simulink model "IDTmodel"  (R2021a)
settings: Solver=ode23tb  StartTime=0.0  StopTime=0.75  FixedStep=4e-4  RelTol=1e-3  EnableMultiTasking=on
PreLoadFcn:
  | % -- Recommended Settings --
  | %
  | %  Simulink:
  | %      Solver: Ode23tb
  | %      Relative tolerance = 1e-4
  | %      Max step size = 0.2
  | %
  | %  Powergui:
  |          Ts = 1e-06; % (discrete electrical model)
  | %
  | %  Control systems:
  |          Ts_control = 10*Ts; % (discrete control system)
  | %
  | % ----------------------------------
InitFcn:
  | Ts=1e-5;
  | Ts_control=1e-5;
undefined symbols (not defined in the file or in its folder): D1, Delta
libraries: spsThreePhaseVIMeasurementLib x26, spsThreePhaseSeriesRLCLoadLib x8, spsabctoAlphaBetaZeroLib x6, spsThreePhaseSeriesRLCBranchLib x6, spsThreePhaseTransformerTwoWindingsLib x5, spsDistributedParametersLineLib x5, spsPowerPositiveSequenceLib x4, spsThreePhaseBreakerLib x4, spsDCVoltageSourceLib x2, spsSVPWMGenerator2LevelLib x2, spsGroundLib x2, spsUniversalBridgeLib x2
(part 1 of 2)
settings Model: Creator=Basit Bukhari  LastModifiedBy=Dell
settings DataIOCC: InitialState=x0  LimitDataPoints=on  ReturnWorkspaceOutputs=off  Refine=10
settings OptimizationCC: EfficientMapNaN2IntZero=off  LifeSpan=inf
settings DebuggingCC: UnconnectedInputMsg=none  UnconnectedOutputMsg=none  UnconnectedLineMsg=none  AllowSymbolicDim=off  SFUnexpectedBacktrackingDiag=warning  SFNoUnconditionalDefaultTransitionDiag=warning  SFExecutionAtInitializationDiag=none  SFMachineParentedDataDiag=warning  ArithmeticOperatorsInVariantConditions=warning
settings HardwareCC: TargetBitPerPointer=64  TargetBitPerSizeT=64  TargetBitPerPtrDiffT=64  TargetLongLongMode=on  TargetIntDivRoundTo=Zero  TargetEndianess=LittleEndian  TargetWordSize=64  TargetHWDeviceType=MATLAB Host  ProdEqTarget=off
settings SFSimCC: SimUseLocalCustomCode=off  CustomCodeUndefinedFunction=UseInterfaceOnly
settings RTWCC: RTWUseLocalCustomCode=off
settings CodeAppCC: MaxIdLength=128
settings GRTTargetCC: TargetLangStandard=C89/C90 (ANSI)  CombineOutputUpdateFcns=off  GRTInterface=on
settings ConfigComp: CovMetricSettings=dw  CovSaveCumulativeToWorkspaceVar=on  CovSaveSingleToWorkspaceVar=on  CovExternalEMLEnable=off  CovSFcnEnable=off
settings SimscapeCC: SimscapeNormalizeSystem=off

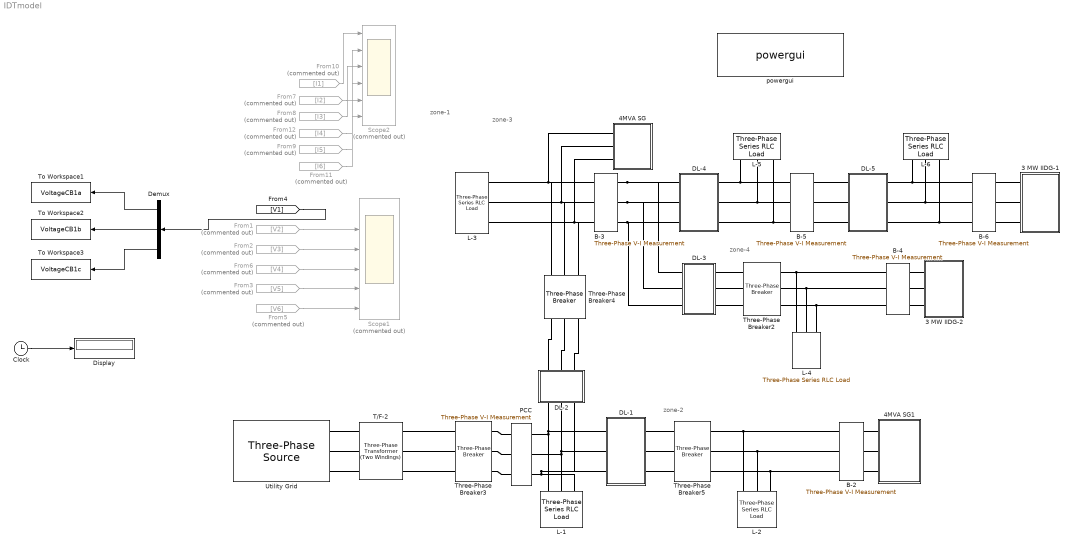
== system IDTmodel ==
  note: zone-2
  note: zone-3
  note: zone-1
  note: zone-4
  " B-2" : spsThreePhaseVIMeasurementLib/Three-Phase V-I Measurement  VoltageMeasurement=phase-to-ground  SetLabelV=on  LabelV=V2  Vpu=on  VpuLL=off  CurrentMeasurement=yes  SetLabelI=on  LabelI=I2  Ipu=on  Pbase=10e6  Vbase=25e3  OutputType=Magnitude  PhasorSimulation=off  PSBequivalent=0
  " B-3" : spsThreePhaseVIMeasurementLib/Three-Phase V-I Measurement  VoltageMeasurement=phase-to-ground  SetLabelV=on  LabelV=V3  Vpu=on  VpuLL=off  CurrentMeasurement=yes  SetLabelI=on  LabelI=I3  Ipu=on  Pbase=10e6  Vbase=25e3  OutputType=Magnitude  PhasorSimulation=off  PSBequivalent=0
  " B-4" : spsThreePhaseVIMeasurementLib/Three-Phase V-I Measurement  VoltageMeasurement=phase-to-ground  SetLabelV=on  LabelV=V4  Vpu=on  VpuLL=off  CurrentMeasurement=yes  SetLabelI=on  LabelI=I4  Ipu=on  Pbase=10e6  Vbase=25e3  OutputType=Magnitude  PhasorSimulation=off  PSBequivalent=0
  " B-5" : spsThreePhaseVIMeasurementLib/Three-Phase V-I Measurement  VoltageMeasurement=phase-to-ground  SetLabelV=on  LabelV=V5  Vpu=on  VpuLL=off  CurrentMeasurement=yes  SetLabelI=on  LabelI=I5  Ipu=on  Pbase=10e6  Vbase=25e3  OutputType=Magnitude  PhasorSimulation=off  PSBequivalent=0
  " B-6" : spsThreePhaseVIMeasurementLib/Three-Phase V-I Measurement  VoltageMeasurement=phase-to-ground  SetLabelV=on  LabelV=V6  Vpu=on  VpuLL=off  CurrentMeasurement=yes  SetLabelI=on  LabelI=I6  Ipu=on  Pbase=10e6  Vbase=25e3  OutputType=Magnitude  PhasorSimulation=off  PSBequivalent=0
  " PCC" : spsThreePhaseVIMeasurementLib/Three-Phase V-I Measurement  VoltageMeasurement=phase-to-ground  SetLabelV=on  LabelV=V1  Vpu=on  VpuLL=off  CurrentMeasurement=yes  SetLabelI=on  LabelI=I1  Ipu=on  Pbase=10e6  Vbase=25e3  OutputType=Magnitude  PhasorSimulation=off  PSBequivalent=0
  3 MW IIDG-1 : Subsystem
  3 MW IIDG-2 : Subsystem
  4MVA SG : Subsystem
  4MVA SG1 : Subsystem
  Clock : Clock
  DL-1 : Subsystem
  DL-2 : Subsystem
  DL-3 : Subsystem
  DL-4 : Subsystem
  DL-5 : Subsystem
  Demux : Demux  Outputs=3
  Display : Display
  From1 : From  Commented=on  GotoTag=V2  TagVisibility=global
  From10 : From  Commented=on  GotoTag=I1  TagVisibility=global
  From11 : From  Commented=on  GotoTag=I6  TagVisibility=global
  From12 : From  Commented=on  GotoTag=I4  TagVisibility=global
  From2 : From  Commented=on  GotoTag=V3  TagVisibility=global
  From3 : From  Commented=on  GotoTag=V5  TagVisibility=global
  From5 : From  Commented=on  GotoTag=V6  TagVisibility=global
  From6 : From  Commented=on  GotoTag=V4  TagVisibility=global
  From7 : From  Commented=on  GotoTag=I2  TagVisibility=global
  From8 : From  Commented=on  GotoTag=I3  TagVisibility=global
  From9 : From  Commented=on  GotoTag=I5  TagVisibility=global
  L-1 : spsThreePhaseSeriesRLCLoadLib/Three-Phase Series RLC Load  LConnTagsString=A|B|C  Configuration=Y (grounded)  NominalVoltage=25e3  Vabc=[7.2 7.2 7.2]*1e3  Vabcp=[1e3 1e3 1e3]  NominalFrequency=50  UnbalancedPower=off  ActivePower=1.5e6  InductivePower=0.6e6  CapacitivePower=0  Pabc=[250 300 350]*1e3  QLabc=[136 170 220]*1e3  QCabc=[0 0 0]  Pabcp=[10e3 9e3 11e3]  QLabcp=[100 90 110]  QCabcp=[100 90 110]  Measurements=None  LoadType=constant PQ
  L-2 : spsThreePhaseSeriesRLCLoadLib/Three-Phase Series RLC Load  LConnTagsString=A|B|C  Configuration=Y (grounded)  NominalVoltage=25e3  Vabc=[7.2 7.2 7.2]*1e3  Vabcp=[1e3 1e3 1e3]  NominalFrequency=50  UnbalancedPower=off  ActivePower=1.5e6  InductivePower=0.3e6  CapacitivePower=0  Pabc=[250 300 350]*1e3  QLabc=[136 170 220]*1e3  QCabc=[0 0 0]  Pabcp=[10e3 9e3 11e3]  QLabcp=[100 90 110]  QCabcp=[100 90 110]  Measurements=None  LoadType=constant PQ
  L-3 : spsThreePhaseSeriesRLCLoadLib/Three-Phase Series RLC Load  LConnTagsString=A|B|C  Configuration=Y (grounded)  NominalVoltage=25e3  Vabc=[7.2 7.2 7.2]*1e3  Vabcp=[1e3 1e3 1e3]  NominalFrequency=50  UnbalancedPower=off  ActivePower=1e6  InductivePower=0.2e6  CapacitivePower=0  Pabc=[250 300 350]*1e3  QLabc=[136 170 220]*1e3  QCabc=[0 0 0]  Pabcp=[10e3 9e3 11e3]  QLabcp=[100 90 110]  QCabcp=[100 90 110]  Measurements=None  LoadType=constant Z
  L-4 : spsThreePhaseSeriesRLCLoadLib/Three-Phase Series RLC Load  LConnTagsString=A|B|C  Configuration=Y (grounded)  NominalVoltage=25e3  Vabc=[7.2 7.2 7.2]*1e3  Vabcp=[1e3 1e3 1e3]  NominalFrequency=50  UnbalancedPower=off  ActivePower=1.5e6  InductivePower=0.6e6  CapacitivePower=0  Pabc=[250 300 350]*1e3  QLabc=[136 170 220]*1e3  QCabc=[0 0 0]  Pabcp=[10e3 9e3 11e3]  QLabcp=[100 90 110]  QCabcp=[100 90 110]  Measurements=None  LoadType=constant Z
  L-5 : spsThreePhaseSeriesRLCLoadLib/Three-Phase Series RLC Load  LConnTagsString=A|B|C  Configuration=Y (grounded)  NominalVoltage=25e3  Vabc=[7.2 7.2 7.2]*1e3  Vabcp=[1e3 1e3 1e3]  NominalFrequency=50  UnbalancedPower=off  ActivePower=0.5e6  InductivePower=0.1e6  CapacitivePower=0  Pabc=[250 300 350]*1e3  QLabc=[136 170 220]*1e3  QCabc=[0 0 0]  Pabcp=[10e3 9e3 11e3]  QLabcp=[100 90 110]  QCabcp=[100 90 110]  Measurements=None  LoadType=constant Z
  L-6 : spsThreePhaseSeriesRLCLoadLib/Three-Phase Series RLC Load  LConnTagsString=A|B|C  Configuration=Y (grounded)  NominalVoltage=25e3  Vabc=[7.2 7.2 7.2]*1e3  Vabcp=[1e3 1e3 1e3]  NominalFrequency=50  UnbalancedPower=off  ActivePower=1e6  InductivePower=0.3e6  CapacitivePower=0  Pabc=[250 300 350]*1e3  QLabc=[136 170 220]*1e3  QCabc=[0 0 0]  Pabcp=[10e3 9e3 11e3]  QLabcp=[100 90 110]  QCabcp=[100 90 110]  Measurements=None  LoadType=constant Z
  Scope1 : Scope  Commented=on  NumInputPorts=6
  Scope2 : Scope  Commented=on  NumInputPorts=6
  T/F-2 : spsThreePhaseTransformerTwoWindingsLib/Three-Phase Transformer (Two Windings)  Winding1Connection=Delta (D1)  Winding2Connection=Yg  CoreType=Three single-phase transformers  SetSaturation=off  Hysteresis=off  DataFile='hysteresis'  SetInitialFlux=off  Measurements=None  UNITS=pu  NominalPower=[20e6 , 50 ]  Winding1=[120e3 , 0.00375 , 0.1]  Winding2=[25e3 , 0.00375 , 0.1]  Rm=500  Lm=500  L0=0.5  Saturation=[ 0,0 ; 0.0024,1.2 ; 1.0,1.52 ]  InitialFluxes=[ 0.8 , -0.8 , 0.7 ]  BreakLoop=off  DiscreteSolver=Trapezoidal iterative  DataType=off  TransfoNumber=1
  Three-Phase Breaker{2..5} (4 alike) : spsThreePhaseBreakerLib/Three-Phase Breaker  InitialState=closed  SwitchA=on  SwitchB=on  SwitchC=on  SwitchTimes=[5]  External=off  BreakerResistance=0.01  SnubberResistance=1e6  SnubberCapacitance=inf  Measurements=None
  To Workspace1 : ToWorkspace  VariableName=VoltageCB1a  SaveFormat=Timeseries  SampleTime=1/3840
  To Workspace2 : ToWorkspace  VariableName=VoltageCB1b  SaveFormat=Timeseries  SampleTime=1/3840
  To Workspace3 : ToWorkspace  VariableName=VoltageCB1c  SaveFormat=Timeseries  SampleTime=1/3840
  "Utility Grid  " : spsThreePhaseSourceLib/Three-Phase Source  InternalConnection=Yg  VoltagePhases=off  Voltage=120e3  PhaseAngle=0  Voltage_phases=[25e3 25e3 25e3]/sqrt(3)  PhaseAngles_phases=[0 -120 +120]  Frequency=50  NonIdealSource=on  SpecifyImpedance=on  Resistance=0.8929  Inductance=16.58e-3  ShortCircuitLevel=500e6  BaseVoltage=120e3  XRratio=7  BusType=swing  Pref=10e6  Qref=5e6  Prefabc=[10e3, 10e3, 10e3]  Qrefabc=[0, 0, 0]  Qmin=-inf  Qmax=inf
  powergui : spspowerguiLib/powergui  Priority=1  SimulationMode=Discrete  SampleTime=10e-6  frequency=60  Iterations=50  frequencyindice=50  Pbase=100e6  ErrMax=1e-4  UnitsV=kV  UnitsW=MW  buscounter=0  FunctionMessages=off  echomessages=off  EnableUseOfTLC=off  CurrentSourceSwitches=off  DisableSnubberDevices=off  DisableRonSwitches=off  DisableVfSwitches=off  DisplayEquations=off  AutomaticDiscreteSolvers=off  SolverType=Tustin/Backward Euler (TBE)  Interpol=off  ExternalGateDelay=off  methode=off  Ts=100  x0status=steady  SPID=on  SwTol=0  HookPort=off  NonlinearTolerance=1e-4  nMaxIteration=100  ContinueOnMaxIteration=off  RestoreLinks=warning  ResistiveCurrentMeasurement=off  Frange=[0:2:500]  Ylog=off  Xlog=on  ShowGrid=off  save=off  variable=ZData  structure=0  ZoomFFT=off  StartTime=0.0  cycles=1  DisplayStyle=1  fundamental=60  FreqAxis=off  MaxFrequency=1000  frequencyindicesteady=1  RmsSteady=1  display=off
  wires:
  From9/1 -> Scope2/5
  From8/1 -> Scope2/3
  From7/1 -> Scope2/2
  From10/1 -> Scope2/1
  From12/1 -> Scope2/4
  From11/1 -> Scope2/6
  Demux/2 -> To Workspace2/1
  Demux/1 -> To Workspace1/1
  Demux/3 -> To Workspace3/1
  From3/1 -> Scope1/5
  From2/1 -> Scope1/3
  From6/1 -> Scope1/4
  [V1] -> Demux/1
  From5/1 -> Scope1/6
  From1/1 -> Scope1/2
  Clock/1 -> Display/1
  connections:
  T/F-2/LConn1 -- "Utility Grid  "/RConn1
  T/F-2/LConn2 -- "Utility Grid  "/RConn2
  T/F-2/LConn3 -- "Utility Grid  "/RConn3
  Three-Phase Breaker3/LConn1 -- T/F-2/RConn1
  Three-Phase Breaker3/LConn2 -- T/F-2/RConn2
  Three-Phase Breaker3/LConn3 -- T/F-2/RConn3
  " PCC"/LConn1 -- Three-Phase Breaker3/RConn1
  " PCC"/LConn2 -- Three-Phase Breaker3/RConn2
  " PCC"/LConn3 -- Three-Phase Breaker3/RConn3
  L-3/LConn1 -- Three-Phase Breaker4/RConn1 -- " B-3"/LConn1 -- 4MVA SG/LConn1
  L-3/LConn2 -- Three-Phase Breaker4/RConn2 -- " B-3"/LConn2 -- 4MVA SG/LConn2
  L-3/LConn3 -- Three-Phase Breaker4/RConn3 -- " B-3"/LConn3 -- 4MVA SG/LConn3
  " PCC"/RConn3 -- L-1/LConn3 -- DL-2/RConn3 -- DL-1/RConn3
  L-1/LConn2 -- DL-2/RConn2 -- DL-1/RConn2 -- " PCC"/RConn2
  L-1/LConn1 -- DL-2/RConn1 -- DL-1/RConn1 -- " PCC"/RConn1
  Three-Phase Breaker5/RConn1 -- " B-2"/RConn1 -- L-2/LConn1
  Three-Phase Breaker5/RConn2 -- " B-2"/RConn2 -- L-2/LConn2
  Three-Phase Breaker5/RConn3 -- " B-2"/RConn3 -- L-2/LConn3
  " B-3"/RConn1 -- DL-3/RConn1 -- DL-4/RConn1
  " B-3"/RConn2 -- DL-3/RConn2 -- DL-4/RConn2
  " B-3"/RConn3 -- DL-3/RConn3 -- DL-4/RConn3
  " B-5"/LConn1 -- DL-4/LConn1 -- L-5/LConn1
  " B-5"/LConn2 -- DL-4/LConn2 -- L-5/LConn2
  " B-5"/LConn3 -- DL-4/LConn3 -- L-5/LConn3
  DL-5/RConn1 -- " B-5"/RConn1
  DL-5/RConn2 -- " B-5"/RConn2
  DL-5/RConn3 -- " B-5"/RConn3
  " B-6"/LConn1 -- DL-5/LConn1 -- L-6/LConn1
  " B-6"/LConn2 -- DL-5/LConn2 -- L-6/LConn2
  " B-6"/LConn3 -- DL-5/LConn3 -- L-6/LConn3
  DL-3/LConn1 -- Three-Phase Breaker2/LConn1
  DL-3/LConn2 -- Three-Phase Breaker2/LConn2
  DL-3/LConn3 -- Three-Phase Breaker2/LConn3
  Three-Phase Breaker2/RConn1 -- " B-4"/LConn1 -- L-4/LConn1
  Three-Phase Breaker2/RConn2 -- L-4/LConn2 -- " B-4"/LConn2
  Three-Phase Breaker2/RConn3 -- L-4/LConn3 -- " B-4"/LConn3
  DL-2/LConn1 -- Three-Phase Breaker4/LConn1
  DL-2/LConn2 -- Three-Phase Breaker4/LConn2
  DL-2/LConn3 -- Three-Phase Breaker4/LConn3
  DL-1/LConn1 -- Three-Phase Breaker5/LConn1
  DL-1/LConn2 -- Three-Phase Breaker5/LConn2
  DL-1/LConn3 -- Three-Phase Breaker5/LConn3
  3 MW IIDG-2/RConn1 -- " B-4"/RConn1
  3 MW IIDG-2/RConn2 -- " B-4"/RConn2
  3 MW IIDG-2/RConn3 -- " B-4"/RConn3
  3 MW IIDG-1/RConn1 -- " B-6"/RConn1
  3 MW IIDG-1/RConn2 -- " B-6"/RConn2
  3 MW IIDG-1/RConn3 -- " B-6"/RConn3
  4MVA SG1/LConn1 -- " B-2"/LConn1
  4MVA SG1/LConn2 -- " B-2"/LConn2
  4MVA SG1/LConn3 -- " B-2"/LConn3

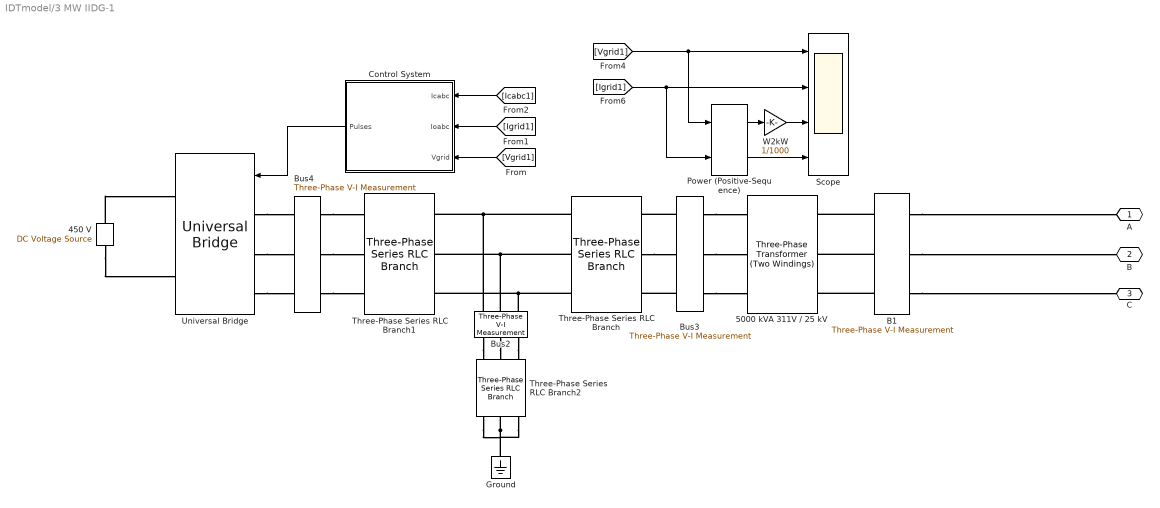
== system IDTmodel/3 MW IIDG-1 ==
  "450 V    " : spsDCVoltageSourceLib/DC Voltage Source  Amplitude=650  Measurements=None
  5000 kVA 311V / 25 kV : spsThreePhaseTransformerTwoWindingsLib/Three-Phase Transformer (Two Windings)  Winding1Connection=Yg  Winding2Connection=Delta (D1)  CoreType=Three single-phase transformers  SetSaturation=off  Hysteresis=off  DataFile='hysteresis'  SetInitialFlux=off  Measurements=None  UNITS=pu  NominalPower=[5e6 , 50 ]  Winding1=[25000 0.001 0.003]  Winding2=[311 0.001 0.003]  Rm=500  Lm=500  L0=0.5  Saturation=[0 0;0.0024 1.2;1 1.52]  InitialFluxes=[0.8 -0.8 0.7]  BreakLoop=off  DiscreteSolver=Trapezoidal iterative  DataType=off  TransfoNumber=0
  B1 : spsThreePhaseVIMeasurementLib/Three-Phase V-I Measurement  VoltageMeasurement=phase-to-ground  SetLabelV=on  LabelV=Vgrid1  Vpu=off  VpuLL=off  CurrentMeasurement=yes  SetLabelI=on  LabelI=Igrid1  Ipu=off  Pbase=100e6  Vbase=500e3  OutputType=Magnitude  PhasorSimulation=off  PSBequivalent=0
  Bus2 : spsThreePhaseVIMeasurementLib/Three-Phase V-I Measurement  VoltageMeasurement=no  SetLabelV=on  LabelV=Vg  Vpu=off  VpuLL=off  CurrentMeasurement=yes  SetLabelI=on  LabelI=Icabc1  Ipu=off  Pbase=100e6  Vbase=500e3  OutputType=Complex  PhasorSimulation=off  PSBequivalent=0
  Bus3 : spsThreePhaseVIMeasurementLib/Three-Phase V-I Measurement  VoltageMeasurement=phase-to-ground  SetLabelV=on  LabelV=Voabc1  Vpu=off  VpuLL=off  CurrentMeasurement=yes  SetLabelI=on  LabelI=Ioabc1  Ipu=off  Pbase=100e6  Vbase=500e3  OutputType=Complex  PhasorSimulation=off  PSBequivalent=0
  Bus4 : spsThreePhaseVIMeasurementLib/Three-Phase V-I Measurement  VoltageMeasurement=phase-to-ground  SetLabelV=on  LabelV=V_inv1  Vpu=off  VpuLL=off  CurrentMeasurement=yes  SetLabelI=on  LabelI=Iinv1  Ipu=off  Pbase=100e6  Vbase=500e3  OutputType=Complex  PhasorSimulation=off  PSBequivalent=0
  Control System : Subsystem
  Ground : spsGroundLib/Ground  LConnTagsString=a
  Power (Positive-Sequence) : spsPowerPositiveSequenceLib/Power (Positive-Sequence)  Freq=50  Vinit=[0, 0]  Iinit=[0, 0]  Ts=10e-6
      settings: SourceProductBaseCode=PS
  Scope : Scope  NumInputPorts=4
  Three-Phase Series RLC Branch : spsThreePhaseSeriesRLCBranchLib/Three-Phase Series RLC Branch  LConnTagsString=A|B|C  RConnTagsString=A|B|C  BranchType=L  Resistance=1  Inductance=0.09e-6  Capacitance=1e-6  Measurements=None
  Three-Phase Series RLC Branch1 : spsThreePhaseSeriesRLCBranchLib/Three-Phase Series RLC Branch  LConnTagsString=A|B|C  RConnTagsString=A|B|C  BranchType=L  Resistance=1e-5  Inductance=8e-5  Capacitance=1e-6  Measurements=None
  Three-Phase Series RLC Branch2 : spsThreePhaseSeriesRLCBranchLib/Three-Phase Series RLC Branch  LConnTagsString=A|B|C  RConnTagsString=A|B|C  BranchType=RC  Resistance=0.005  Inductance=1e-3  Capacitance=0.0041  Measurements=None
  Universal Bridge : spsUniversalBridgeLib/Universal Bridge  Arms=3  SnubberResistance=1e5  SnubberCapacitance=inf  Device=IGBT / Diodes  Ron=1e-3  Lon=0  ForwardVoltages="[  0  0  ]"  ForwardVoltage=0  GTOparameters=[ 10e-6 , 20e-6 ]  IGBTparameters=[ 1e-6 , 2e-6 ]  Measurements=None  Measurements_2=None  converterType=Rectifier
  W2kW : Gain  Gain=1/1000
  A : PMIOPort  Side=Right
  B : PMIOPort  Port=2  Side=Right
  C : PMIOPort  Port=3  Side=Right
  wires:
  [Igrid1] -> Control System/2(Ioabc)
  Control System/1(Pulses) -> Universal Bridge/1
  [Vgrid1] -> Control System/3(Vgrid)
  [Icabc1] -> Control System/1(Icabc)
  Power (Positive-Sequence)/1 -> W2kW/1
  [Igrid1] -> Scope/2, Power (Positive-Sequence)/2
  [Vgrid1] -> Scope/1, Power (Positive-Sequence)/1
  W2kW/1 -> Scope/3
  Power (Positive-Sequence)/2 -> Scope/4
  connections:
  Universal Bridge/LConn2 -- Bus4/LConn2
  Bus3/RConn3 -- 5000 kVA 311V / 25 kV/RConn3
  B1/LConn1 -- 5000 kVA 311V / 25 kV/LConn1
  Three-Phase Series RLC Branch/RConn2 -- Bus3/LConn2
  "450 V    "/LConn1 -- Universal Bridge/RConn2
  Bus3/LConn3 -- Three-Phase Series RLC Branch/RConn3
  Bus3/RConn1 -- 5000 kVA 311V / 25 kV/RConn1
  B1/LConn3 -- 5000 kVA 311V / 25 kV/LConn3
  B1/LConn2 -- 5000 kVA 311V / 25 kV/LConn2
  Universal Bridge/LConn1 -- Bus4/LConn1
  Bus3/LConn1 -- Three-Phase Series RLC Branch/RConn1
  Bus4/RConn1 -- Three-Phase Series RLC Branch1/LConn1
  Bus4/RConn2 -- Three-Phase Series RLC Branch1/LConn2
  Universal Bridge/LConn3 -- Bus4/LConn3
  Bus2/RConn3 -- Three-Phase Series RLC Branch2/LConn3
  Bus3/RConn2 -- 5000 kVA 311V / 25 kV/RConn2
  Bus2/RConn2 -- Three-Phase Series RLC Branch2/LConn2
  Bus4/RConn3 -- Three-Phase Series RLC Branch1/LConn3
  Bus2/RConn1 -- Three-Phase Series RLC Branch2/LConn1
  "450 V    "/RConn1 -- Universal Bridge/RConn1
  Bus2/LConn2 -- Three-Phase Series RLC Branch/LConn2 -- Three-Phase Series RLC Branch1/RConn2
  Three-Phase Series RLC Branch2/RConn2 -- Ground/LConn1 -- Three-Phase Series RLC Branch2/RConn1 -- Three-Phase Series RLC Branch2/RConn3
  Bus2/LConn3 -- Three-Phase Series RLC Branch/LConn3 -- Three-Phase Series RLC Branch1/RConn3
  Bus2/LConn1 -- Three-Phase Series RLC Branch/LConn1 -- Three-Phase Series RLC Branch1/RConn1
  B1/RConn2 -- B/RConn1
  B1/RConn1 -- A/RConn1
  B1/RConn3 -- C/RConn1

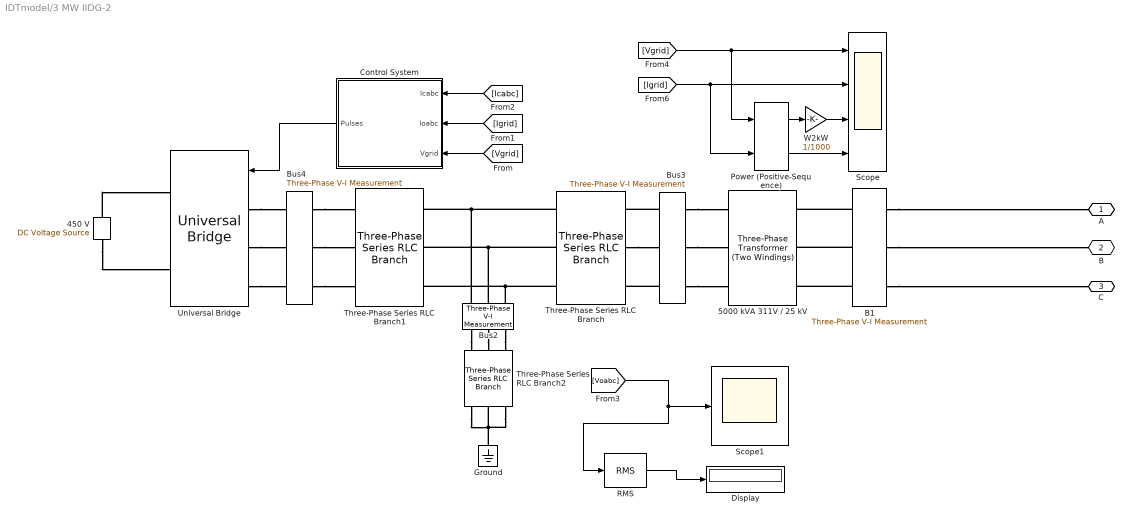
== system IDTmodel/3 MW IIDG-2 ==
  "450 V    " : spsDCVoltageSourceLib/DC Voltage Source  Amplitude=650  Measurements=None
  5000 kVA 311V / 25 kV : spsThreePhaseTransformerTwoWindingsLib/Three-Phase Transformer (Two Windings)  Winding1Connection=Yg  Winding2Connection=Delta (D1)  CoreType=Three single-phase transformers  SetSaturation=off  Hysteresis=off  DataFile='hysteresis'  SetInitialFlux=off  Measurements=None  UNITS=pu  NominalPower=[5e6 , 50 ]  Winding1=[25000 0.001 0.003]  Winding2=[311 0.001 0.003]  Rm=500  Lm=500  L0=0.5  Saturation=[0 0;0.0024 1.2;1 1.52]  InitialFluxes=[0.8 -0.8 0.7]  BreakLoop=off  DiscreteSolver=Trapezoidal iterative  DataType=off  TransfoNumber=0
  B1 : spsThreePhaseVIMeasurementLib/Three-Phase V-I Measurement  VoltageMeasurement=phase-to-ground  SetLabelV=on  LabelV=Vgrid  Vpu=off  VpuLL=off  CurrentMeasurement=yes  SetLabelI=on  LabelI=Igrid  Ipu=off  Pbase=100e6  Vbase=500e3  OutputType=Magnitude  PhasorSimulation=off  PSBequivalent=0
  Bus2 : spsThreePhaseVIMeasurementLib/Three-Phase V-I Measurement  VoltageMeasurement=no  SetLabelV=on  LabelV=Vg  Vpu=off  VpuLL=off  CurrentMeasurement=yes  SetLabelI=on  LabelI=Icabc  Ipu=off  Pbase=100e6  Vbase=500e3  OutputType=Complex  PhasorSimulation=off  PSBequivalent=0
  Bus3 : spsThreePhaseVIMeasurementLib/Three-Phase V-I Measurement  VoltageMeasurement=phase-to-ground  SetLabelV=on  LabelV=Voabc  Vpu=off  VpuLL=off  CurrentMeasurement=yes  SetLabelI=on  LabelI=Ioabc  Ipu=off  Pbase=100e6  Vbase=500e3  OutputType=Complex  PhasorSimulation=off  PSBequivalent=0
  Bus4 : spsThreePhaseVIMeasurementLib/Three-Phase V-I Measurement  VoltageMeasurement=phase-to-ground  SetLabelV=on  LabelV=V_inv  Vpu=off  VpuLL=off  CurrentMeasurement=yes  SetLabelI=on  LabelI=Iinv  Ipu=off  Pbase=100e6  Vbase=500e3  OutputType=Complex  PhasorSimulation=off  PSBequivalent=0
  Control System : Subsystem
  Display : Display
  Ground : spsGroundLib/Ground  LConnTagsString=a
  Power (Positive-Sequence) : spsPowerPositiveSequenceLib/Power (Positive-Sequence)  Freq=50  Vinit=[0, 0]  Iinit=[0, 0]  Ts=10e-6
      settings: SourceProductBaseCode=PS
  RMS : spsRMSLib/RMS  TrueRMS=on  Freq=60  RMSInit=120  Ts=0
  Scope : Scope  NumInputPorts=4
  Scope1 : Scope
  Three-Phase Series RLC Branch : spsThreePhaseSeriesRLCBranchLib/Three-Phase Series RLC Branch  LConnTagsString=A|B|C  RConnTagsString=A|B|C  BranchType=L  Resistance=1  Inductance=0.09e-6  Capacitance=1e-6  Measurements=None
  Three-Phase Series RLC Branch1 : spsThreePhaseSeriesRLCBranchLib/Three-Phase Series RLC Branch  LConnTagsString=A|B|C  RConnTagsString=A|B|C  BranchType=L  Resistance=1e-5  Inductance=8e-5  Capacitance=1e-6  Measurements=None
  Three-Phase Series RLC Branch2 : spsThreePhaseSeriesRLCBranchLib/Three-Phase Series RLC Branch  LConnTagsString=A|B|C  RConnTagsString=A|B|C  BranchType=RC  Resistance=0.005  Inductance=1e-3  Capacitance=0.0041  Measurements=None
  Universal Bridge : spsUniversalBridgeLib/Universal Bridge  Arms=3  SnubberResistance=1e5  SnubberCapacitance=inf  Device=IGBT / Diodes  Ron=1e-3  Lon=0  ForwardVoltages="[  0  0  ]"  ForwardVoltage=0  GTOparameters=[ 10e-6 , 20e-6 ]  IGBTparameters=[ 1e-6 , 2e-6 ]  Measurements=None  Measurements_2=None  converterType=Rectifier
  W2kW : Gain  Gain=1/1000
  A : PMIOPort  Side=Right
  B : PMIOPort  Port=2  Side=Right
  C : PMIOPort  Port=3  Side=Right
  wires:
  W2kW/1 -> Scope/3
  Power (Positive-Sequence)/2 -> Scope/4
  [Igrid] -> Scope/2, Power (Positive-Sequence)/2
  Power (Positive-Sequence)/1 -> W2kW/1
  [Vgrid] -> Scope/1, Power (Positive-Sequence)/1
  [Icabc] -> Control System/1(Icabc)
  [Vgrid] -> Control System/3(Vgrid)
  Control System/1(Pulses) -> Universal Bridge/1
  [Igrid] -> Control System/2(Ioabc)
  [Voabc] -> RMS/1, Scope1/1
  RMS/1 -> Display/1
  connections:
  B1/RConn3 -- C/RConn1
  B1/RConn1 -- A/RConn1
  B1/RConn2 -- B/RConn1
  Three-Phase Series RLC Branch/LConn1 -- Bus2/LConn1 -- Three-Phase Series RLC Branch1/RConn1
  Three-Phase Series RLC Branch/LConn3 -- Bus2/LConn3 -- Three-Phase Series RLC Branch1/RConn3
  Ground/LConn1 -- Three-Phase Series RLC Branch2/RConn2 -- Three-Phase Series RLC Branch2/RConn3 -- Three-Phase Series RLC Branch2/RConn1
  Three-Phase Series RLC Branch/LConn2 -- Bus2/LConn2 -- Three-Phase Series RLC Branch1/RConn2
  "450 V    "/RConn1 -- Universal Bridge/RConn1
  Bus2/RConn1 -- Three-Phase Series RLC Branch2/LConn1
  Bus4/RConn3 -- Three-Phase Series RLC Branch1/LConn3
  Bus2/RConn2 -- Three-Phase Series RLC Branch2/LConn2
  Bus3/RConn2 -- 5000 kVA 311V / 25 kV/RConn2
  Bus2/RConn3 -- Three-Phase Series RLC Branch2/LConn3
  Universal Bridge/LConn3 -- Bus4/LConn3
  Bus4/RConn2 -- Three-Phase Series RLC Branch1/LConn2
  Bus4/RConn1 -- Three-Phase Series RLC Branch1/LConn1
  Bus3/LConn1 -- Three-Phase Series RLC Branch/RConn1
  Universal Bridge/LConn1 -- Bus4/LConn1
  B1/LConn2 -- 5000 kVA 311V / 25 kV/LConn2
  B1/LConn3 -- 5000 kVA 311V / 25 kV/LConn3
  Bus3/RConn1 -- 5000 kVA 311V / 25 kV/RConn1
  Bus3/LConn3 -- Three-Phase Series RLC Branch/RConn3
  "450 V    "/LConn1 -- Universal Bridge/RConn2
  Three-Phase Series RLC Branch/RConn2 -- Bus3/LConn2
  B1/LConn1 -- 5000 kVA 311V / 25 kV/LConn1
  Bus3/RConn3 -- 5000 kVA 311V / 25 kV/RConn3
  Universal Bridge/LConn2 -- Bus4/LConn2

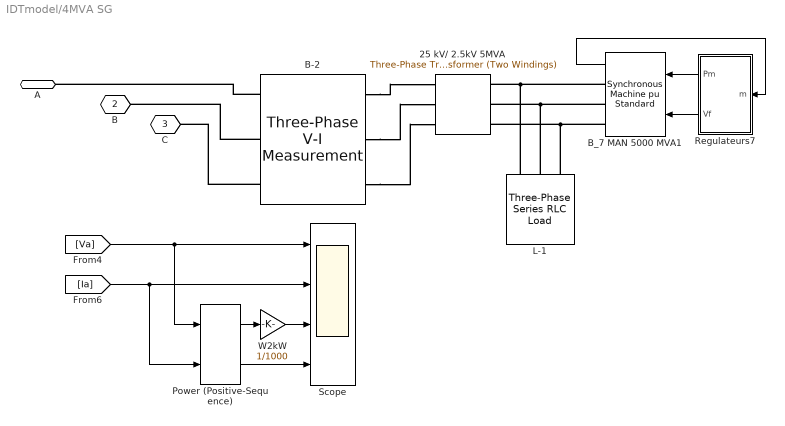
== system IDTmodel/4MVA SG ==
  " B-2" : spsThreePhaseVIMeasurementLib/Three-Phase V-I Measurement  VoltageMeasurement=phase-to-ground  SetLabelV=on  LabelV=Va  Vpu=off  VpuLL=off  CurrentMeasurement=yes  SetLabelI=on  LabelI=Ia  Ipu=off  Pbase=10e6  Vbase=25e3  OutputType=Magnitude  PhasorSimulation=off  PSBequivalent=0
  25 kV/ 2.5kV 5MVA : spsThreePhaseTransformerTwoWindingsLib/Three-Phase Transformer (Two Windings)  Winding1Connection=Delta (D1)  Winding2Connection=Yg  CoreType=Three-limb core (core-type)  SetSaturation=off  Hysteresis=off  DataFile='hysteresis'  SetInitialFlux=off  Measurements=None  UNITS=pu  NominalPower="[5e6  50]"  Winding1=[25e3 , 0.0025 , 0.0025]  Winding2=[2400, 0.0025 , 0.0025]  Rm=500  Lm=500  L0=0.5  Saturation=[ 0,0 ; 0.0024,1.2 ; 1.0,1.52 ]  InitialFluxes=[ 0.8 , -0.8 , 0.7 ]  BreakLoop=off  DiscreteSolver=Trapezoidal iterative  DataType=off  TransfoNumber=0
  B_7 MAN 5000 MVA1 : spsSynchronousMachinepuStandardLib/Synchronous Machine pu Standard  PresetModel=No  MechanicalLoad=Mechanical power Pm  ShowDetailedParameters=on  RotorType=Salient-pole  Units=per unit standard parameters  MeasurementBus=off  NominalParameters="[4E6  2400   50]"  Reactances1=[2.16 0.47 0.22 2 0.85 0.25 0.2]  Reactances2=[1.6 0.47 0.22 2 0.75 0.85 0.3]  dAxisTimeConstants=Short-circuit  qAxisTimeConstants=Open-circuit  TimeConstants1=0.041 0.06 0.058 0.056]  TimeConstants2=[0.075 0.068 0.019 0.015]  TimeConstants3=[ 0.05, 0.053, 0.01 ]  TimeConstants4=[]  TimeConstants5=[0.052 0.03 0.03]  TimeConstants6=[]  TimeConstants7=[0.000052 0.00003 0.00003]  TimeConstants8=[]  StatorResistance=0.009  Mechanical=[25 0 1]  PolePairs=32  InitialConditions=[0 22.0414 0.903015 0.903015 0.903015 48.7213 -71.2787 168.721 1.8534]  SetSaturation=off  Saturation=[0.6404,0.7127,0.8441,0.9214,0.9956,1.082,1.19,1.316,1.457;0.7,0.7698,0.8872,0.9466,0.9969,1.046,1.1,1.151,1.201]  LoadFlowParameters=[4 3500000 0 0 500000]  TsPowergui=0  TsBlock=-1  IterativeModel=Trapezoidal non iterative  IterativeDiscreteModel=Trapezoidal iterative (alg. loop)  BusType=PQ  Pref=3.5e6  Qref=0.5e6  Qmin=-Inf  Qmax=Inf  PLF=0  QLF=0
      settings: SourceProductBaseCode=PS
  L-1 : spsThreePhaseSeriesRLCLoadLib/Three-Phase Series RLC Load  LConnTagsString=A|B|C  Configuration=Y (grounded)  NominalVoltage=2.4e3  Vabc=[7.2 7.2 7.2]*1e3  Vabcp=[1e3 1e3 1e3]  NominalFrequency=50  UnbalancedPower=off  ActivePower=5e3  InductivePower=0  CapacitivePower=0  Pabc=[250 300 350]*1e3  QLabc=[136 170 220]*1e3  QCabc=[0 0 0]  Pabcp=[10e3 9e3 11e3]  QLabcp=[100 90 110]  QCabcp=[100 90 110]  Measurements=None  LoadType=constant PQ
  Power (Positive-Sequence) : spsPowerPositiveSequenceLib/Power (Positive-Sequence)  Freq=50  Vinit=[0, 0]  Iinit=[0, 0]  Ts=10e-6
      settings: SourceProductBaseCode=PS
  Regulateurs7 : Subsystem
  Scope : Scope  NumInputPorts=4
  W2kW : Gain  Gain=1/1000
  A : PMIOPort  Tag=PMCPort  Side=Left
  B : PMIOPort  Tag=PMCPort  Port=2  Side=Left
  C : PMIOPort  Tag=PMCPort  Port=3  Side=Left
  wires:
  Power (Positive-Sequence)/2 -> Scope/4
  Power (Positive-Sequence)/1 -> W2kW/1
  W2kW/1 -> Scope/3
  [Va] -> Scope/1, Power (Positive-Sequence)/1
  [Ia] -> Scope/2, Power (Positive-Sequence)/2
  Regulateurs7/1(Pm) -> B_7 MAN 5000 MVA1/1
  B_7 MAN 5000 MVA1/1 -> Regulateurs7/1(m)
  Regulateurs7/2(Vf) -> B_7 MAN 5000 MVA1/2
  connections:
  L-1/LConn3 -- B_7 MAN 5000 MVA1/RConn3 -- 25 kV/ 2.5kV 5MVA/RConn3
  L-1/LConn1 -- B_7 MAN 5000 MVA1/RConn1 -- 25 kV/ 2.5kV 5MVA/RConn1
  L-1/LConn2 -- B_7 MAN 5000 MVA1/RConn2 -- 25 kV/ 2.5kV 5MVA/RConn2
  " B-2"/RConn3 -- C/RConn1
  " B-2"/RConn2 -- B/RConn1
  " B-2"/RConn1 -- A/RConn1
  " B-2"/LConn1 -- 25 kV/ 2.5kV 5MVA/LConn1
  " B-2"/LConn2 -- 25 kV/ 2.5kV 5MVA/LConn2
  " B-2"/LConn3 -- 25 kV/ 2.5kV 5MVA/LConn3

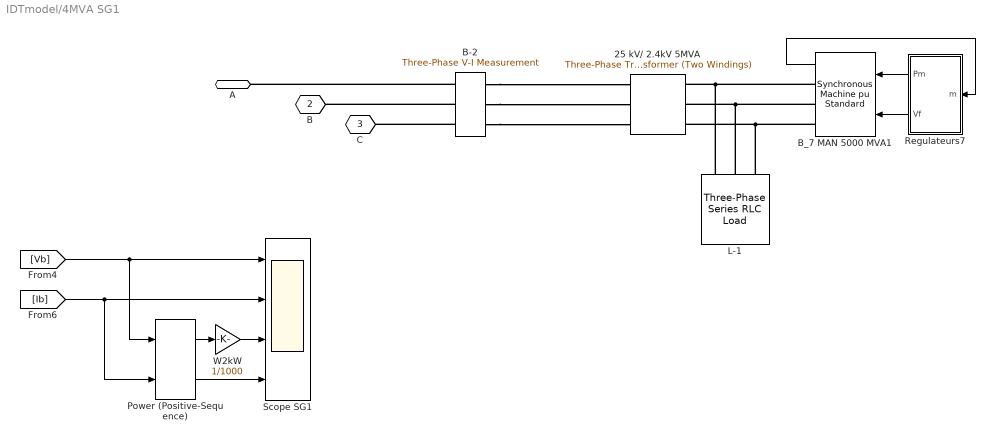
== system IDTmodel/4MVA SG1 ==
  " B-2" : spsThreePhaseVIMeasurementLib/Three-Phase V-I Measurement  VoltageMeasurement=phase-to-ground  SetLabelV=on  LabelV=Vb  Vpu=off  VpuLL=off  CurrentMeasurement=yes  SetLabelI=on  LabelI=Ib  Ipu=off  Pbase=10e6  Vbase=25e3  OutputType=Magnitude  PhasorSimulation=off  PSBequivalent=0
  25 kV/ 2.4kV 5MVA : spsThreePhaseTransformerTwoWindingsLib/Three-Phase Transformer (Two Windings)  Winding1Connection=Delta (D1)  Winding2Connection=Yg  CoreType=Three-limb core (core-type)  SetSaturation=off  Hysteresis=off  DataFile='hysteresis'  SetInitialFlux=off  Measurements=None  UNITS=pu  NominalPower="[5e6  50]"  Winding1=[25e3 , 0.0025 , 0.0025]  Winding2=[2400, 0.0025 , 0.0025]  Rm=500  Lm=500  L0=0.5  Saturation=[ 0,0 ; 0.0024,1.2 ; 1.0,1.52 ]  InitialFluxes=[ 0.8 , -0.8 , 0.7 ]  BreakLoop=off  DiscreteSolver=Trapezoidal iterative  DataType=off  TransfoNumber=0
  B_7 MAN 5000 MVA1 : spsSynchronousMachinepuStandardLib/Synchronous Machine pu Standard  PresetModel=No  MechanicalLoad=Mechanical power Pm  ShowDetailedParameters=on  RotorType=Salient-pole  Units=per unit standard parameters  MeasurementBus=off  NominalParameters="[4E6  2400   50]"  Reactances1=[2.16 0.47 0.22 2 0.85 0.25 0.2]  Reactances2=[1.6 0.47 0.22 2 0.75 0.85 0.3]  dAxisTimeConstants=Short-circuit  qAxisTimeConstants=Open-circuit  TimeConstants1=0.041 0.06 0.058 0.056]  TimeConstants2=[0.075 0.068 0.019 0.015]  TimeConstants3=[ 0.05, 0.053, 0.01 ]  TimeConstants4=[]  TimeConstants5=[0.052 0.03 0.03]  TimeConstants6=[]  TimeConstants7=[0.000052 0.00003 0.00003]  TimeConstants8=[]  StatorResistance=0.009  Mechanical=[25 0 1]  PolePairs=32  InitialConditions=[0 22.7829 0.892432 0.892432 0.892432 49.9645 -70.0355 169.964 1.84636]  SetSaturation=off  Saturation=[0.6404,0.7127,0.8441,0.9214,0.9956,1.082,1.19,1.316,1.457;0.7,0.7698,0.8872,0.9466,0.9969,1.046,1.1,1.151,1.201]  LoadFlowParameters=[4 3500000 0 0 500000]  TsPowergui=0  TsBlock=-1  IterativeModel=Trapezoidal non iterative  IterativeDiscreteModel=Trapezoidal iterative (alg. loop)  BusType=PQ  Pref=3.5e6  Qref=0.5e6  Qmin=-Inf  Qmax=Inf  PLF=0  QLF=0
      settings: SourceProductBaseCode=PS
  L-1 : spsThreePhaseSeriesRLCLoadLib/Three-Phase Series RLC Load  LConnTagsString=A|B|C  Configuration=Y (grounded)  NominalVoltage=2.4e3  Vabc=[7.2 7.2 7.2]*1e3  Vabcp=[1e3 1e3 1e3]  NominalFrequency=50  UnbalancedPower=off  ActivePower=100  InductivePower=0  CapacitivePower=0  Pabc=[250 300 350]*1e3  QLabc=[136 170 220]*1e3  QCabc=[0 0 0]  Pabcp=[10e3 9e3 11e3]  QLabcp=[100 90 110]  QCabcp=[100 90 110]  Measurements=None  LoadType=constant PQ
  Power (Positive-Sequence) : spsPowerPositiveSequenceLib/Power (Positive-Sequence)  Freq=60  Vinit=[0, 0]  Iinit=[0, 0]  Ts=10e-6
      settings: SourceProductBaseCode=PS
  Regulateurs7 : Subsystem
  Scope SG1 : Scope  NumInputPorts=4
  W2kW : Gain  Gain=1/1000
  A : PMIOPort  Tag=PMCPort  Side=Left
  B : PMIOPort  Tag=PMCPort  Port=2  Side=Left
  C : PMIOPort  Tag=PMCPort  Port=3  Side=Left
  wires:
  Power (Positive-Sequence)/2 -> Scope SG1/4
  Power (Positive-Sequence)/1 -> W2kW/1
  W2kW/1 -> Scope SG1/3
  [Vb] -> Scope SG1/1, Power (Positive-Sequence)/1
  [Ib] -> Scope SG1/2, Power (Positive-Sequence)/2
  Regulateurs7/1(Pm) -> B_7 MAN 5000 MVA1/1
  B_7 MAN 5000 MVA1/1 -> Regulateurs7/1(m)
  Regulateurs7/2(Vf) -> B_7 MAN 5000 MVA1/2
  connections:
  L-1/LConn3 -- B_7 MAN 5000 MVA1/RConn3 -- 25 kV/ 2.4kV 5MVA/RConn3
  L-1/LConn1 -- B_7 MAN 5000 MVA1/RConn1 -- 25 kV/ 2.4kV 5MVA/RConn1
  L-1/LConn2 -- B_7 MAN 5000 MVA1/RConn2 -- 25 kV/ 2.4kV 5MVA/RConn2
  " B-2"/RConn3 -- C/RConn1
  " B-2"/RConn2 -- B/RConn1
  " B-2"/RConn1 -- A/RConn1
  " B-2"/LConn1 -- 25 kV/ 2.4kV 5MVA/LConn1
  " B-2"/LConn2 -- 25 kV/ 2.4kV 5MVA/LConn2
  " B-2"/LConn3 -- 25 kV/ 2.4kV 5MVA/LConn3

== system IDTmodel/DL-1 ==
  20Km feeder : spsDistributedParametersLineLib/Distributed Parameters Line  Phases=3  Length=20  Frequency=50  Resistance=[0.1153 0.413]  Inductance=[1.05e-3 3.32e-3]  Capacitance=[11.33e-009 5.01e-009]  x1=[-9e-05 -2.68516105709753e-09 0 0;-8e-05 -2.68300659765662e-09 0 0;-7e-05 -2.68082565802377e-09 21285.8674089973 -12894.4169654849;-6e-05 -2.67861825972396e-09 21326.2713065149 -12827.4819194618;-5e-05 -2.67638442454334e-09 21366.4647223445 -12760.4202713709;-4e-05 -2.67412417452894e-09 21406.4472597932 -12693.2326830835;-3e-05 -2.67183753198853e-09 21446.2185242496 -12625.9198177139;-2e-05 -2.66952451949035e-09 21485.7781231874 -12558.4823396131;-1e-05 -2.66718515986289e-09 21525.1256661693 -12490.9209143616]  x2=[-9e-05 -1.81112936076848e-08 0 0;-8e-05 -1.81037637267218e-08 0 0;-7e-05 -1.80960551689196e-08 21779.6080777928 -12619.3778514325;-6e-05 -1.80881680103586e-08 21819.1454793611 -12550.8930331657;-5e-05 -1.80801023288818e-08 21858.4675347722 -12482.2843426516;-4e-05 -1.80718582040943e-08 21897.5738559334 -12413.5524570303;-3e-05 -1.80634357173622e-08 21936.4640568811 -12344.6980546578;-2e-05 -1.8054834951812e-08 21975.1377537846 -12275.7218150993;-1e-05 -1.804605599233e-08 22013.5945649502 -12206.6244191224]  x3=[-9e-05 -3.24823942318317e-10 0 0;-8e-05 -3.26732084948908e-10 0 0;-7e-05 -3.28637002865727e-10 129.304247380407 -96.3808150004817;-6e-05 -3.30538677268004e-10 129.606398052337 -95.9741187751671;-5e-05 -3.32437089386981e-10 129.907269561442 -95.5664753240466;-4e-05 -3.34332220486095e-10 130.206858938243 -95.1578886703963;-3e-05 -3.36224051861169e-10 130.505163225913 -94.7483628468017;-2e-05 -3.3811256484059e-10 130.802179480308 -94.3379018951172;-1e-05 -3.39997740785497e-10 131.097904769999 -93.9265098664268]  x4=[-9e-05 2.99120956574791e-10 0 0;-8e-05 3.01038609687328e-10 0 0;-7e-05 3.02953291670321e-10 10.4549897173436 11.5184203719103;-6e-05 3.04864983626632e-10 10.4187519987774 11.5512087956851;-5e-05 3.06773666688634e-10 10.3824114513352 11.5838832136926;-4e-05 3.08679322018396e-10 10.3459684336836 11.6164433034493;-3e-05 3.10581930807868e-10 10.3094233055003 11.6488887436004;-2e-05 3.1248147427907e-10 10.272776427471 11.6812192139224;-1e-05 3.14377933684274e-10 10.2360281612858 11.7134343953267]  x5=8.1567640642598e-05  V1=[0 0 0 8.565e-09 2.497e+04 2.497e+04;0 0 0 314.2 314.2 314.2;1.571 1.571 1.571 2.095 1.026 -0.545]  V2=[0 0 0 4.522e-08 2.525e+04 2.525e+04;0 0 0 314.2 314.2 314.2;1.571 1.571 1.571 1.876 1.045 -0.5256]  I1=[0 0 0 1.638e-09 161.4 161.4;0 0 0 314.2 314.2 314.2;1.571 1.571 1.571 0.6386 0.9308 -0.64]  I2=[0 0 0 1.619e-09 15.51 15.51;0 0 0 314.2 314.2 314.2;1.571 1.571 1.571 -2.542 2.375 0.8038]  nHarmo=2  Measurements=None  Decoupling=off  VsMag0=0  VrMag0=0  VsAngle0=0  VrAngle0=0  IsMag0=0  IrMag0=0  IsAngle0=0  IrAngle0=0
      settings: SourceProductBaseCode=PS
  Three-Phase V-I Measurement1 : spsThreePhaseVIMeasurementLib/Three-Phase V-I Measurement  VoltageMeasurement=no  SetLabelV=off  LabelV=Vabc  Vpu=on  VpuLL=off  CurrentMeasurement=no  SetLabelI=off  LabelI=I23  Ipu=on  Pbase=6e6  Vbase=12.47e3  OutputType=Complex  PhasorSimulation=off  PSBequivalent=0
  Three-Phase V-I Measurement4 : spsThreePhaseVIMeasurementLib/Three-Phase V-I Measurement  VoltageMeasurement=no  SetLabelV=off  LabelV=Vabc  Vpu=on  VpuLL=off  CurrentMeasurement=no  SetLabelI=off  LabelI=I23  Ipu=on  Pbase=6e6  Vbase=12.47e3  OutputType=Complex  PhasorSimulation=off  PSBequivalent=0
  Three-Phase Fault : spsThreePhaseFaultLib/Three-Phase Fault  InitialStates=0  FaultA=on  FaultB=on  FaultC=off  GroundFault=on  SwitchTimes=[0.5]  External=off  SwitchStatus=NaN  FaultResistance=R  GroundResistance=0.01  SnubberResistance=1e6  SnubberCapacitance=inf  Measurements=None
  A : PMIOPort  Side=Right
  B : PMIOPort  Port=2  Side=Right
  C : PMIOPort  Port=3  Side=Right
  a : PMIOPort  Port=4  Side=Left
  b : PMIOPort  Port=5  Side=Left
  c : PMIOPort  Port=6  Side=Left
  connections:
  20Km feeder/RConn2 -- Three-Phase V-I Measurement1/RConn2
  20Km feeder/RConn1 -- Three-Phase V-I Measurement1/RConn1
  20Km feeder/RConn3 -- Three-Phase V-I Measurement1/RConn3
  20Km feeder/LConn3 -- Three-Phase Fault/LConn3 -- Three-Phase V-I Measurement4/RConn3
  20Km feeder/LConn2 -- Three-Phase Fault/LConn2 -- Three-Phase V-I Measurement4/RConn2
  20Km feeder/LConn1 -- Three-Phase Fault/LConn1 -- Three-Phase V-I Measurement4/RConn1
  C/RConn1 -- Three-Phase V-I Measurement4/LConn3
  B/RConn1 -- Three-Phase V-I Measurement4/LConn2
  A/RConn1 -- Three-Phase V-I Measurement4/LConn1
  b/RConn1 -- Three-Phase V-I Measurement1/LConn2
  a/RConn1 -- Three-Phase V-I Measurement1/LConn1
  c/RConn1 -- Three-Phase V-I Measurement1/LConn3

== system IDTmodel/DL-2 ==
  20Km feeder : spsDistributedParametersLineLib/Distributed Parameters Line  Phases=3  Length=20  Frequency=50  Resistance=[0.1153 0.413]  Inductance=[1.05e-3 3.32e-3]  Capacitance=[11.33e-009 5.01e-009]  x1=[-9e-05 -2.68510963323614e-09 0 0;-8e-05 -2.6829608862793e-09 0 0;-7e-05 -2.68078565958166e-09 21285.8674089973 -12894.4169654849;-6e-05 -2.67858397461185e-09 21326.2713065149 -12827.4819194618;-5e-05 -2.67635585309959e-09 21366.4647223445 -12760.4202713709;-4e-05 -2.67410131703555e-09 21406.4472597932 -12693.2326830835;-3e-05 -2.67182038867109e-09 21446.2185242497 -12625.9198177139;-2e-05 -2.66951309051805e-09 21485.7781231874 -12558.4823396131;-1e-05 -2.66717944534854e-09 21525.1256661693 -12490.9209143616]  x2=[-9e-05 2.73721764290198e-09 0 0;-8e-05 2.73130177773865e-09 0 0;-7e-05 2.72535895572945e-09 21166.2455226375 -12931.8216327417;-6e-05 2.71938923552763e-09 21206.7675204995 -12865.2622047554;-5e-05 2.71339267605191e-09 21247.0802161276 -12798.575801825;-4e-05 2.70736933648592e-09 21287.1832116518 -12731.7630821185;-3e-05 2.70131927627759e-09 21327.0761112717 -12664.8247050504;-2e-05 2.69524255513857e-09 21366.7585212604 -12597.7613312755;-1e-05 2.68913923304365e-09 21406.2300499687 -12530.5736226821]  x3=[-9e-05 1.9043730135867e-10 0 0;-8e-05 1.91009282245078e-10 0 0;-7e-05 1.91579377946985e-10 58.4084045621915 -28.5327517806663;-6e-05 1.92147582837774e-10 58.4977544644372 -28.3491158644527;-5e-05 1.92713891309495e-10 58.5865270174628 -28.1652001539106;-4e-05 1.9327829777291e-10 58.674721345119 -27.9810064642138;-3e-05 1.93840796657555e-10 58.7623365769635 -27.7965366132795;-2e-05 1.94401382411794e-10 58.8493718482694 -27.6117924217507;-1e-05 1.94960049502872e-10 58.9358263000335 -27.4267757129781]  x4=[-9e-05 -1.90931896511564e-10 0 0;-8e-05 -1.91508640277674e-10 0 0;-7e-05 -1.9208349393082e-10 79.3363379225984 -57.3284218242058;-6e-05 -1.92656451797428e-10 79.5160486663739 -57.0788968736236;-5e-05 -1.93227508222635e-10 79.6949746188509 -56.8288085773731;-4e-05 -1.93796657570345e-10 79.8731140141027 -56.5781594037245;-3e-05 -1.94363894223284e-10 80.0504650939652 -56.3269518264842;-2e-05 -1.94929212583055e-10 80.2270261080548 -56.0751883249695;-1e-05 -1.95492607070194e-10 80.4027953137858 -55.8228713839844]  x5=8.1567640642598e-05  V1=[0 0 0 8.564e-09 2.497e+04 2.497e+04;0 0 0 314.2 314.2 314.2;1.571 1.571 1.571 2.094 1.026 -0.545]  V2=[0 0 0 2.195e-09 2.496e+04 2.496e+04;0 0 0 314.2 314.2 314.2;1.571 1.571 1.571 2.087 1.021 -0.5502]  I1=[0 0 0 2.786e-10 63.92 63.92;0 0 0 314.2 314.2 314.2;1.571 1.571 1.571 -2.274 0.9423 -0.6285]  I2=[0 0 0 2.832e-10 99.42 99.42;0 0 0 314.2 314.2 314.2;1.571 1.571 1.571 0.9124 1.057 -0.5134]  nHarmo=2  Measurements=None  Decoupling=off  VsMag0=0  VrMag0=0  VsAngle0=0  VrAngle0=0  IsMag0=0  IrMag0=0  IsAngle0=0  IrAngle0=0
      settings: SourceProductBaseCode=PS
  Three-Phase V-I Measurement1 : spsThreePhaseVIMeasurementLib/Three-Phase V-I Measurement  VoltageMeasurement=no  SetLabelV=off  LabelV=Vabc  Vpu=on  VpuLL=off  CurrentMeasurement=no  SetLabelI=off  LabelI=I23  Ipu=on  Pbase=6e6  Vbase=12.47e3  OutputType=Complex  PhasorSimulation=off  PSBequivalent=0
  Three-Phase V-I Measurement4 : spsThreePhaseVIMeasurementLib/Three-Phase V-I Measurement  VoltageMeasurement=no  SetLabelV=off  LabelV=Vabc  Vpu=on  VpuLL=off  CurrentMeasurement=no  SetLabelI=off  LabelI=I23  Ipu=on  Pbase=6e6  Vbase=12.47e3  OutputType=Complex  PhasorSimulation=off  PSBequivalent=0
  A : PMIOPort  Side=Right
  B : PMIOPort  Port=2  Side=Right
  C : PMIOPort  Port=3  Side=Right
  a : PMIOPort  Port=4  Side=Left
  b : PMIOPort  Port=5  Side=Left
  c : PMIOPort  Port=6  Side=Left
  connections:
  c/RConn1 -- Three-Phase V-I Measurement1/LConn3
  a/RConn1 -- Three-Phase V-I Measurement1/LConn1
  b/RConn1 -- Three-Phase V-I Measurement1/LConn2
  A/RConn1 -- Three-Phase V-I Measurement4/LConn1
  B/RConn1 -- Three-Phase V-I Measurement4/LConn2
  C/RConn1 -- Three-Phase V-I Measurement4/LConn3
  20Km feeder/LConn1 -- Three-Phase V-I Measurement4/RConn1
  20Km feeder/LConn2 -- Three-Phase V-I Measurement4/RConn2
  20Km feeder/LConn3 -- Three-Phase V-I Measurement4/RConn3
  20Km feeder/RConn3 -- Three-Phase V-I Measurement1/RConn3
  20Km feeder/RConn1 -- Three-Phase V-I Measurement1/RConn1
  20Km feeder/RConn2 -- Three-Phase V-I Measurement1/RConn2

== system IDTmodel/DL-3 ==
  20Km feeder : spsDistributedParametersLineLib/Distributed Parameters Line  Phases=3  Length=20  Frequency=50  Resistance=[0.1153 0.413]  Inductance=[1.05e-3 3.32e-3]  Capacitance=[11.33e-009 5.01e-009]  x1=[-9e-05 -3.54138350635367e-09 0 0;-8e-05 -3.53568235282156e-09 0 0;-7e-05 -3.52994630353204e-09 21166.1431215582 -12931.6701657764;-6e-05 -3.52417541509761e-09 21206.6646440788 -12865.1110602396;-5e-05 -3.51836974447459e-09 21246.976865381 -12798.4249812504;-4e-05 -3.51252934896262e-09 21287.0793875992 -12731.6125869736;-3e-05 -3.50665428620404e-09 21326.9718149377 -12664.6745368205;-2e-05 -3.50074461418335e-09 21366.6537536745 -12597.6114914427;-1e-05 -3.49480039122663e-09 21406.1248121649 -12530.4241127253]  x2=[-9e-05 -1.49165436309215e-10 0 0;-8e-05 -1.49069334365799e-10 0 0;-7e-05 -1.48971761168235e-10 20762.5558966759 -13090.3392509388;-6e-05 -1.4887271767953e-10 20803.5778836304 -13025.0472669771;-5e-05 -1.48772204877205e-10 20844.39454767 -12959.6267310574;-4e-05 -1.48670223753279e-10 20885.0054859505 -12894.0782888539;-3e-05 -1.48566775314265e-10 20925.4102976586 -12828.4025873032;-2e-05 -1.48461860581157e-10 20965.6085840149 -12762.6002745979;-1e-05 -1.48355480589422e-10 21005.5999482787 -12696.6720001805]  x3=[-9e-05 1.24071467571665e-10 0 0;-8e-05 1.24425361907173e-10 0 0;-7e-05 1.24778028214592e-10 28.3409315330498 3.86101835923995;-6e-05 1.25129463013247e-10 28.3286619493135 3.950034821736;-5e-05 1.25479662834619e-10 28.3161127731204 4.03901229898306;-4e-05 1.25828624222377e-10 28.3032841283259 4.12794991280934;-3e-05 1.26176343732413e-10 28.2901761415436 4.2168467854365;-2e-05 1.26522817932875e-10 28.276788942144 4.3057020394883;-1e-05 1.26868043404204e-10 28.2631226622533 4.39451479799925]  x4=[-9e-05 -1.28650202189275e-10 0 0;-8e-05 -1.28997804169447e-10 0 0;-7e-05 -1.29344132993371e-10 107.687251309224 -90.3430738276636;-6e-05 -1.29689185242921e-10 107.97054056455 -90.0043190817292;-5e-05 -1.3003295751257e-10 108.25276419423 -89.6646760295017;-4e-05 -1.30375446409425e-10 108.533919412831 -89.3241480231209;-3e-05 -1.30716648553258e-10 108.814003445464 -88.9827384234607;-2e-05 -1.31056560576543e-10 109.093013527813 -88.640450600096;-1e-05 -1.31395179124484e-10 109.370946906161 -88.2972879312695]  x5=8.1567640642598e-05  V1=[0 0 0 3.967e-09 2.496e+04 2.496e+04;0 0 0 314.2 314.2 314.2;1.571 1.571 1.571 2.209 1.021 -0.5502]  V2=[0 0 0 1.223e-10 2.477e+04 2.477e+04;0 0 0 314.2 314.2 314.2;1.571 1.571 1.571 3.034 1.005 -0.5654]  I1=[0 0 0 1.709e-10 22.9 22.9;0 0 0 314.2 314.2 314.2;1.571 1.571 1.571 -2.176 1.307 -0.2639]  I2=[0 0 0 1.723e-10 140.8 140.8;0 0 0 314.2 314.2 314.2;1.571 1.571 1.571 0.9925 0.9534 -0.6174]  nHarmo=2  Measurements=None  Decoupling=off  VsMag0=0  VrMag0=0  VsAngle0=0  VrAngle0=0  IsMag0=0  IrMag0=0  IsAngle0=0  IrAngle0=0
      settings: SourceProductBaseCode=PS
  Three-Phase V-I Measurement1 : spsThreePhaseVIMeasurementLib/Three-Phase V-I Measurement  VoltageMeasurement=no  SetLabelV=off  LabelV=Vabc  Vpu=on  VpuLL=off  CurrentMeasurement=no  SetLabelI=off  LabelI=I23  Ipu=on  Pbase=6e6  Vbase=12.47e3  OutputType=Complex  PhasorSimulation=off  PSBequivalent=0
  Three-Phase V-I Measurement4 : spsThreePhaseVIMeasurementLib/Three-Phase V-I Measurement  VoltageMeasurement=no  SetLabelV=off  LabelV=Vabc  Vpu=on  VpuLL=off  CurrentMeasurement=no  SetLabelI=off  LabelI=I23  Ipu=on  Pbase=6e6  Vbase=12.47e3  OutputType=Complex  PhasorSimulation=off  PSBequivalent=0
  A : PMIOPort  Side=Right
  B : PMIOPort  Port=2  Side=Right
  C : PMIOPort  Port=3  Side=Right
  a : PMIOPort  Port=4  Side=Left
  b : PMIOPort  Port=5  Side=Left
  c : PMIOPort  Port=6  Side=Left
  connections:
  20Km feeder/RConn2 -- Three-Phase V-I Measurement1/RConn2
  20Km feeder/RConn1 -- Three-Phase V-I Measurement1/RConn1
  20Km feeder/RConn3 -- Three-Phase V-I Measurement1/RConn3
  20Km feeder/LConn3 -- Three-Phase V-I Measurement4/RConn3
  20Km feeder/LConn2 -- Three-Phase V-I Measurement4/RConn2
  20Km feeder/LConn1 -- Three-Phase V-I Measurement4/RConn1
  C/RConn1 -- Three-Phase V-I Measurement4/LConn3
  B/RConn1 -- Three-Phase V-I Measurement4/LConn2
  A/RConn1 -- Three-Phase V-I Measurement4/LConn1
  b/RConn1 -- Three-Phase V-I Measurement1/LConn2
  a/RConn1 -- Three-Phase V-I Measurement1/LConn1
  c/RConn1 -- Three-Phase V-I Measurement1/LConn3

== system IDTmodel/DL-4 ==
  20Km feeder : spsDistributedParametersLineLib/Distributed Parameters Line  Phases=3  Length=20  Frequency=50  Resistance=[0.1153 0.413]  Inductance=[1.05e-3 3.32e-3]  Capacitance=[11.33e-009 5.01e-009]  x1=[-9e-05 -3.54138350635367e-09 0 0;-8e-05 -3.53568235282156e-09 0 0;-7e-05 -3.52994630353204e-09 21166.1431215582 -12931.6701657764;-6e-05 -3.52417541509761e-09 21206.6646440788 -12865.1110602396;-5e-05 -3.51836974447459e-09 21246.976865381 -12798.4249812504;-4e-05 -3.51252934896262e-09 21287.0793875992 -12731.6125869736;-3e-05 -3.50665428620404e-09 21326.9718149377 -12664.6745368205;-2e-05 -3.50074461418335e-09 21366.6537536745 -12597.6114914427;-1e-05 -3.49480039122663e-09 21406.1248121649 -12530.4241127253]  x2=[-9e-05 -1.85670213466245e-09 0 0;-8e-05 -1.85399954048981e-09 0 0;-7e-05 -1.85127864809018e-09 20803.2327751115 -13139.8661984527;-6e-05 -1.8485394843177e-09 20844.4101545723 -13074.4461801133;-5e-05 -1.84578207620678e-09 20885.3818081202 -13008.8971222685;-4e-05 -1.84300645097195e-09 20926.1473313813 -12943.219671861;-3e-05 -1.8402126360075e-09 20966.7063220166 -12877.4144771007;-2e-05 -1.83740065888725e-09 21007.058379725 -12811.4821874584;-1e-05 -1.83457054736429e-09 21047.2031062481 -12745.4234536591]  x3=[-9e-05 6.21822295601665e-11 0 0;-8e-05 6.23572893617542e-11 0 0;-7e-05 6.25317337220705e-11 23.589010107937 -3.9425127941792;-6e-05 6.27055609194201e-11 23.601279449791 -3.8683863997151;-5e-05 6.28787692381986e-11 23.6133158565449 -3.79422182583897;-4e-05 6.305135696891e-11 23.6251192094045 -3.7200198045252;-3e-05 6.32233224081829e-11 23.6366893918753 -3.6457810681178;-2e-05 6.3394663858788e-11 23.6480262897643 -3.57150634932312;-1e-05 6.35653796296542e-11 23.6591297911809 -3.49719638120264]  x4=[-9e-05 -6.85326073651836e-11 0 0;-8e-05 -6.86993738646141e-11 0 0;-7e-05 -6.88654623289597e-11 112.570278607873 -82.7027540930025;-6e-05 -6.90308711189942e-11 112.829541033579 -82.3486965930491;-5e-05 -6.91955986021997e-11 113.087689877265 -81.9938263447059;-4e-05 -6.93596431527823e-11 113.344722591107 -81.6381468503989;-3e-05 -6.95230031516887e-11 113.600636638297 -81.2816616205411;-2e-05 -6.96856769866215e-11 113.855429493066 -80.9243741734979;-1e-05 -6.98476630520557e-11 114.10909864071 -80.566288035552]  x5=8.1567640642598e-05  V1=[0 0 0 3.967e-09 2.496e+04 2.496e+04;0 0 0 314.2 314.2 314.2;1.571 1.571 1.571 2.209 1.021 -0.5502]  V2=[0 0 0 1.943e-09 2.476e+04 2.476e+04;0 0 0 314.2 314.2 314.2;1.571 1.571 1.571 2.212 1.006 -0.5651]  I1=[0 0 0 8.77e-11 24.06 24.06;0 0 0 314.2 314.2 314.2;1.571 1.571 1.571 -2.181 1.403 -0.1673]  I2=[0 0 0 9.058e-11 140.5 140.5;0 0 0 314.2 314.2 314.2;1.571 1.571 1.571 1.037 0.9354 -0.6354]  nHarmo=2  Measurements=None  Decoupling=off  VsMag0=0  VrMag0=0  VsAngle0=0  VrAngle0=0  IsMag0=0  IrMag0=0  IsAngle0=0  IrAngle0=0
      settings: SourceProductBaseCode=PS
  Three-Phase V-I Measurement1 : spsThreePhaseVIMeasurementLib/Three-Phase V-I Measurement  VoltageMeasurement=no  SetLabelV=off  LabelV=Vabc  Vpu=on  VpuLL=off  CurrentMeasurement=no  SetLabelI=off  LabelI=I23  Ipu=on  Pbase=6e6  Vbase=12.47e3  OutputType=Complex  PhasorSimulation=off  PSBequivalent=0
  Three-Phase V-I Measurement4 : spsThreePhaseVIMeasurementLib/Three-Phase V-I Measurement  VoltageMeasurement=no  SetLabelV=off  LabelV=Vabc  Vpu=on  VpuLL=off  CurrentMeasurement=no  SetLabelI=off  LabelI=I23  Ipu=on  Pbase=6e6  Vbase=12.47e3  OutputType=Complex  PhasorSimulation=off  PSBequivalent=0
  A : PMIOPort  Side=Right
  B : PMIOPort  Port=2  Side=Right
  C : PMIOPort  Port=3  Side=Right
  a : PMIOPort  Port=4  Side=Left
  b : PMIOPort  Port=5  Side=Left
  c : PMIOPort  Port=6  Side=Left
  connections:
  20Km feeder/RConn2 -- Three-Phase V-I Measurement1/RConn2
  20Km feeder/RConn1 -- Three-Phase V-I Measurement1/RConn1
  20Km feeder/RConn3 -- Three-Phase V-I Measurement1/RConn3
  20Km feeder/LConn3 -- Three-Phase V-I Measurement4/RConn3
  20Km feeder/LConn2 -- Three-Phase V-I Measurement4/RConn2
  20Km feeder/LConn1 -- Three-Phase V-I Measurement4/RConn1
  C/RConn1 -- Three-Phase V-I Measurement4/LConn3
  B/RConn1 -- Three-Phase V-I Measurement4/LConn2
  A/RConn1 -- Three-Phase V-I Measurement4/LConn1
  b/RConn1 -- Three-Phase V-I Measurement1/LConn2
  a/RConn1 -- Three-Phase V-I Measurement1/LConn1
  c/RConn1 -- Three-Phase V-I Measurement1/LConn3
